simulink model "Scenario_MinimumExample_TwithTrafficLights_tol"  (R2021a)
settings: Solver=VariableStepAuto  StartTime=0.0  StopTime=50  RelTol=1e-3
model workspace (MAT data in the model file):
  Kz_dif : Simulink.Parameter (value not decoded)
  Kz_il : Simulink.Parameter (value not decoded)
  Kz_ir : Simulink.Parameter (value not decoded)
  Kz_is : Simulink.Parameter (value not decoded)
  Kz_long : Simulink.Parameter (value not decoded)
  Kz_pre : Simulink.Parameter (value not decoded)
  L_dif : Simulink.Parameter (value not decoded)
  L_il : Simulink.Parameter (value not decoded)
  L_ir : Simulink.Parameter (value not decoded)
  L_is : Simulink.Parameter (value not decoded)
  L_long : Simulink.Parameter (value not decoded)
  L_pre : Simulink.Parameter (value not decoded)
  Lc : Simulink.Parameter (value not decoded)
  Rk : Simulink.Parameter (value not decoded)
  Tz_dif : Simulink.Parameter (value not decoded)
  Tz_il : Simulink.Parameter (value not decoded)
  Tz_ir : Simulink.Parameter (value not decoded)
  Tz_is : Simulink.Parameter (value not decoded)
  Tz_long : Simulink.Parameter (value not decoded)
  Tz_pre : Simulink.Parameter (value not decoded)
  ds : Simulink.Parameter (value not decoded)
  dt : Simulink.Parameter (value not decoded)
  v : Simulink.Parameter (value not decoded)
symbols that are objects in the model workspace (value not decoded): Kz_dif, Kz_il, Kz_ir, Kz_is, Kz_long, Kz_pre, Rk, Tz_dif, Tz_il, Tz_ir, Tz_is, Tz_long, Tz_pre
libraries: StreetLanesLibrary x72, EdgesLibrary x64, MeasuringLibrary x33, SourcesAndSinksLibrary x12, LightsLibrary x2
(part 2 of 2)

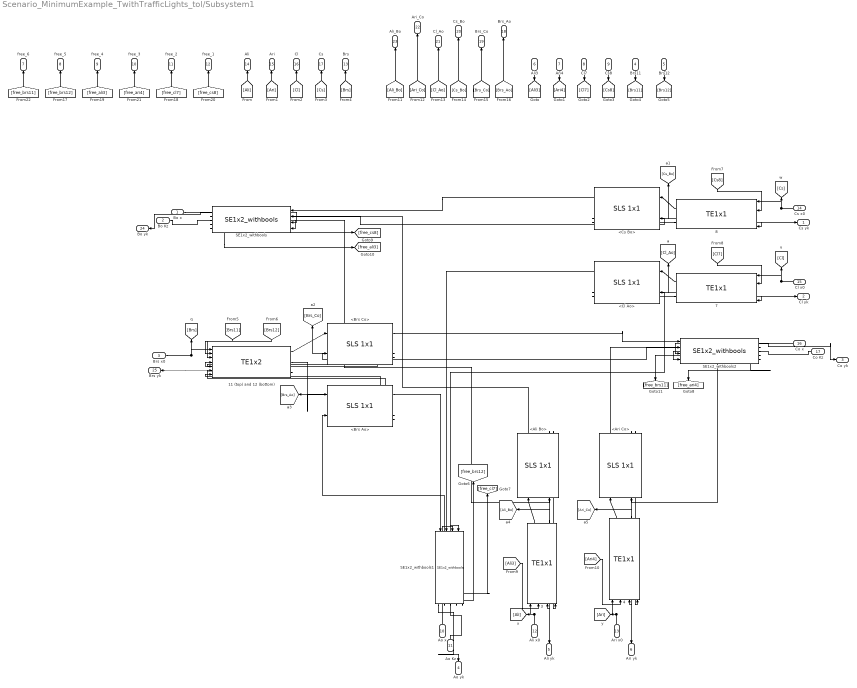
== system Scenario_MinimumExample_TwithTrafficLights_tol/Subsystem1 ==
  Bo x : Inport
  Bo Kz : Inport  Port=2
  Brs x0 : Inport  Port=3
  Brs11 : Inport  Port=4
  Brs12 : Inport  Port=5
  Ali3 : Inport  Port=6
  Ari4 : Inport  Port=7
  Cl7 : Inport  Port=8
  Cs8 : Inport  Port=9
  Ao x : Inport  Port=10
  Ao Kz : Inport  Port=11
  Ali x0 : Inport  Port=12
  Ari x0 : Inport  Port=13
  Cs x0 : Inport  Port=14
  Cl x0 : Inport  Port=15
  Co x : Inport  Port=16
  Co Kz : Inport  Port=17
  11 (top) and 12 (bottom) : EdgesLibrary/TE1x2  Rk1=0.5*Rk  Rk2=0.5*Rk
  {3..4,7..8} (4 alike) : EdgesLibrary/TE1x1  Rk=Rk  slope=2000
  <Ali Bo> : StreetLanesLibrary/SLS 1x1  Kz=Kz_left  Tz=Tz_left
  <Ari Co> : StreetLanesLibrary/SLS 1x1  Kz=Kz_right  Tz=Tz_right
  <Brs Ao> : StreetLanesLibrary/SLS 1x1  Kz=Kz_right  Tz=Tz_right
  <Brs Co> : StreetLanesLibrary/SLS 1x1  Kz=Kz_straight  Tz=Tz_straight
  <Cl Ao> : StreetLanesLibrary/SLS 1x1  Kz=Kz_left  Tz=Tz_left
  <Cs Bo> : StreetLanesLibrary/SLS 1x1  Kz=Kz_straight  Tz=Tz_straight
  SE1x2_withbools : EdgesLibrary/SE1x2_withbools  Rk1=Rk  Rk2=Rk
  SE1x2_withbools1 : EdgesLibrary/SE1x2_withbools  Rk1=Rk  Rk2=Rk
  SE1x2_withbools2 : EdgesLibrary/SE1x2_withbools  Rk1=Rk  Rk2=Rk
  Cs yk : Outport
  Cl yk : Outport  Port=2
  Co yk : Outport  Port=3
  Ao yk : Outport  Port=4
  Ali yk : Outport  Port=5
  Ari yk : Outport  Port=6
  free_6 : Outport  Port=7
  free_5 : Outport  Port=8
  free_4 : Outport  Port=9
  free_3 : Outport  Port=10
  free_2 : Outport  Port=11
  free_1 : Outport  Port=12
  Brs : Outport  Port=13
  Ali : Outport  Port=14
  Ari : Outport  Port=15
  Cl : Outport  Port=16
  Cs : Outport  Port=17
  Brs_Ao : Outport  Port=18
  Brs_Co : Outport  Port=19
  Cs_Bo : Outport  Port=20
  Cl_Ao : Outport  Port=21
  Ari_Co : Outport  Port=22
  Ali_Bo : Outport  Port=23
  Bo yk : Outport  Port=24
  Brs yk : Outport  Port=25
  wires:
  11 (top) and 12 (bottom)/2 -> <Brs Ao>/1
  11 (top) and 12 (bottom)/3 -> Brs yk/1
  3/2 -> Ali yk/1
  3/1 -> <Ali Bo>/1
  Ari x0/1 -> [Ari], 4/1
  <Cs Bo>/2 -> SE1x2_withbools/1
  <Cs Bo>/8 -> 8/4
  <Cl Ao>/8 -> 7/4
  Co x/1 -> SE1x2_withbools2/3
  SE1x2_withbools2/1 -> Co yk/1
  SE1x2_withbools2/3 -> <Ari Co>/2
  <Ari Co>/8 -> 4/4
  <Ali Bo>/8 -> 3/4
  Ao x/1 -> SE1x2_withbools1/3
  Brs x0/1 -> 11 (top) and 12 (bottom)/1, [Brs]
  <Brs Co>/2 -> SE1x2_withbools2/1
  <Cl Ao>/7 -> [Cl_Ao], 7/3
  <Cl Ao>/2 -> SE1x2_withbools1/2
  SE1x2_withbools/2 -> <Cs Bo>/2
  <Ari Co>/2 -> SE1x2_withbools2/2
  7/1 -> <Cl Ao>/1
  Cl x0/1 -> [Cl], 7/1
  4/1 -> <Ari Co>/1
  <Ari Co>/7 -> 4/3, [Ari_Co]
  <Brs Ao>/2 -> SE1x2_withbools1/1
  Ao Kz/1 -> SE1x2_withbools1/4
  <Brs Ao>/7 -> [Brs_Ao], 11 (top) and 12 (bottom)/6
  <Brs Ao>/8 -> 11 (top) and 12 (bottom)/7
  Co Kz/1 -> SE1x2_withbools2/4
  8/2 -> Cs yk/1
  Bo Kz/1 -> SE1x2_withbools/4
  SE1x2_withbools1/3 -> <Cl Ao>/2
  <Brs Co>/8 -> 11 (top) and 12 (bottom)/5
  [Brs12] -> 11 (top) and 12 (bottom)/3
  SE1x2_withbools/3 -> <Ali Bo>/2
  <Ali Bo>/7 -> 3/3, [Ali_Bo]
  SE1x2_withbools1/2 -> <Brs Ao>/2
  Ali x0/1 -> [Ali], 3/1
  <Brs Co>/7 -> 11 (top) and 12 (bottom)/4, [Brs_Co]
  SE1x2_withbools1/1 -> Ao yk/1
  <Ali Bo>/2 -> SE1x2_withbools/2
  [Ari4] -> 4/2
  SE1x2_withbools2/2 -> <Brs Co>/2
  8/1 -> <Cs Bo>/1
  4/2 -> Ari yk/1
  <Cs Bo>/7 -> 8/3, [Cs_Bo]
  Cs x0/1 -> [Cs], 8/1
  [Ali3] -> 3/2
  [Brs11] -> 11 (top) and 12 (bottom)/2
  11 (top) and 12 (bottom)/1 -> <Brs Co>/1
  Bo x/1 -> SE1x2_withbools/3
  [Cl7] -> 7/2
  SE1x2_withbools/1 -> Bo yk/1
  7/2 -> Cl yk/1
  [Cs8] -> 8/2
  [Ali_Bo] -> Ali_Bo/1
  [Ari_Co] -> Ari_Co/1
  [Cl_Ao] -> Cl_Ao/1
  [Cs_Bo] -> Cs_Bo/1
  [Brs_Co] -> Brs_Co/1
  [Brs_Ao] -> Brs_Ao/1
  [Ali] -> Ali/1
  [Ari] -> Ari/1
  [Cl] -> Cl/1
  [Cs] -> Cs/1
  [Brs] -> Brs/1
  Ali3/1 -> [Ali3]
  Ari4/1 -> [Ari4]
  Cl7/1 -> [Cl7]
  Cs8/1 -> [Cs8]
  Brs11/1 -> [Brs11]
  Brs12/1 -> [Brs12]
  SE1x2_withbools1/4 -> [free_brs12]
  SE1x2_withbools1/5 -> [free_cl7]
  SE1x2_withbools/4 -> [free_cs8]
  SE1x2_withbools/5 -> [free_ali3]
  SE1x2_withbools2/5 -> [free_ari4]
  SE1x2_withbools2/4 -> [free_brs11]
  [free_cs8] -> free_1/1
  [free_cl7] -> free_2/1
  [free_ari4] -> free_3/1
  [free_ali3] -> free_4/1
  [free_brs12] -> free_5/1
  [free_brs11] -> free_6/1

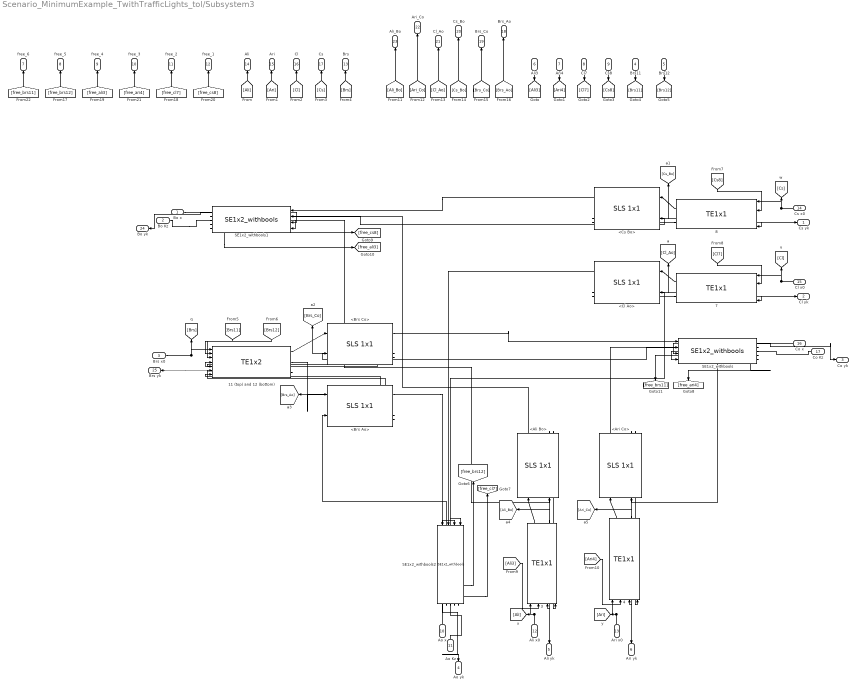
== system Scenario_MinimumExample_TwithTrafficLights_tol/Subsystem3 ==
  Bo x : Inport
  Bo Kz : Inport  Port=2
  Brs x0 : Inport  Port=3
  Brs11 : Inport  Port=4
  Brs12 : Inport  Port=5
  Ali3 : Inport  Port=6
  Ari4 : Inport  Port=7
  Cl7 : Inport  Port=8
  Cs8 : Inport  Port=9
  Ao x : Inport  Port=10
  Ao Kz : Inport  Port=11
  Ali x0 : Inport  Port=12
  Ari x0 : Inport  Port=13
  Cs x0 : Inport  Port=14
  Cl x0 : Inport  Port=15
  Co x : Inport  Port=16
  Co Kz : Inport  Port=17
  11 (top) and 12 (bottom) : EdgesLibrary/TE1x2  Rk1=0.5*Rk  Rk2=0.5*Rk
  {3..4,7..8} (4 alike) : EdgesLibrary/TE1x1  Rk=Rk  slope=2000
  <Ali Bo> : StreetLanesLibrary/SLS 1x1  Kz=Kz_left  Tz=Tz_left
  <Ari Co> : StreetLanesLibrary/SLS 1x1  Kz=Kz_right  Tz=Tz_right
  <Brs Ao> : StreetLanesLibrary/SLS 1x1  Kz=Kz_right  Tz=Tz_right
  <Brs Co> : StreetLanesLibrary/SLS 1x1  Kz=Kz_straight  Tz=Tz_straight
  <Cl Ao> : StreetLanesLibrary/SLS 1x1  Kz=Kz_left  Tz=Tz_left
  <Cs Bo> : StreetLanesLibrary/SLS 1x1  Kz=Kz_straight  Tz=Tz_straight
  SE1x2_withbools : EdgesLibrary/SE1x2_withbools  Rk1=Rk  Rk2=Rk
  SE1x2_withbools1 : EdgesLibrary/SE1x2_withbools  Rk1=Rk  Rk2=Rk
  SE1x2_withbools2 : EdgesLibrary/SE1x2_withbools  Rk1=Rk  Rk2=Rk
  Cs yk : Outport
  Cl yk : Outport  Port=2
  Co yk : Outport  Port=3
  Ao yk : Outport  Port=4
  Ali yk : Outport  Port=5
  Ari yk : Outport  Port=6
  free_6 : Outport  Port=7
  free_5 : Outport  Port=8
  free_4 : Outport  Port=9
  free_3 : Outport  Port=10
  free_2 : Outport  Port=11
  free_1 : Outport  Port=12
  Brs : Outport  Port=13
  Ali : Outport  Port=14
  Ari : Outport  Port=15
  Cl : Outport  Port=16
  Cs : Outport  Port=17
  Brs_Ao : Outport  Port=18
  Brs_Co : Outport  Port=19
  Cs_Bo : Outport  Port=20
  Cl_Ao : Outport  Port=21
  Ari_Co : Outport  Port=22
  Ali_Bo : Outport  Port=23
  Bo yk : Outport  Port=24
  Brs yk : Outport  Port=25
  wires:
  11 (top) and 12 (bottom)/2 -> <Brs Ao>/1
  11 (top) and 12 (bottom)/3 -> Brs yk/1
  3/2 -> Ali yk/1
  3/1 -> <Ali Bo>/1
  Ari x0/1 -> [Ari], 4/1
  <Cs Bo>/2 -> SE1x2_withbools1/1
  <Cs Bo>/8 -> 8/4
  <Cl Ao>/8 -> 7/4
  Co x/1 -> SE1x2_withbools/3
  SE1x2_withbools/1 -> Co yk/1
  SE1x2_withbools/3 -> <Ari Co>/2
  <Ari Co>/8 -> 4/4
  <Ali Bo>/8 -> 3/4
  Ao x/1 -> SE1x2_withbools2/3
  Brs x0/1 -> 11 (top) and 12 (bottom)/1, [Brs]
  <Brs Co>/2 -> SE1x2_withbools/1
  <Cl Ao>/7 -> [Cl_Ao], 7/3
  <Cl Ao>/2 -> SE1x2_withbools2/2
  SE1x2_withbools1/2 -> <Cs Bo>/2
  <Ari Co>/2 -> SE1x2_withbools/2
  7/1 -> <Cl Ao>/1
  Cl x0/1 -> [Cl], 7/1
  4/1 -> <Ari Co>/1
  <Ari Co>/7 -> 4/3, [Ari_Co]
  <Brs Ao>/2 -> SE1x2_withbools2/1
  Ao Kz/1 -> SE1x2_withbools2/4
  <Brs Ao>/7 -> [Brs_Ao], 11 (top) and 12 (bottom)/6
  <Brs Ao>/8 -> 11 (top) and 12 (bottom)/7
  Co Kz/1 -> SE1x2_withbools/4
  8/2 -> Cs yk/1
  Bo Kz/1 -> SE1x2_withbools1/4
  SE1x2_withbools2/3 -> <Cl Ao>/2
  <Brs Co>/8 -> 11 (top) and 12 (bottom)/5
  [Brs12] -> 11 (top) and 12 (bottom)/3
  SE1x2_withbools1/3 -> <Ali Bo>/2
  <Ali Bo>/7 -> 3/3, [Ali_Bo]
  SE1x2_withbools2/2 -> <Brs Ao>/2
  Ali x0/1 -> [Ali], 3/1
  <Brs Co>/7 -> 11 (top) and 12 (bottom)/4, [Brs_Co]
  SE1x2_withbools2/1 -> Ao yk/1
  <Ali Bo>/2 -> SE1x2_withbools1/2
  [Ari4] -> 4/2
  SE1x2_withbools/2 -> <Brs Co>/2
  8/1 -> <Cs Bo>/1
  4/2 -> Ari yk/1
  <Cs Bo>/7 -> 8/3, [Cs_Bo]
  Cs x0/1 -> [Cs], 8/1
  [Ali3] -> 3/2
  [Brs11] -> 11 (top) and 12 (bottom)/2
  11 (top) and 12 (bottom)/1 -> <Brs Co>/1
  Bo x/1 -> SE1x2_withbools1/3
  [Cl7] -> 7/2
  SE1x2_withbools1/1 -> Bo yk/1
  7/2 -> Cl yk/1
  [Cs8] -> 8/2
  [Ali_Bo] -> Ali_Bo/1
  [Ari_Co] -> Ari_Co/1
  [Cl_Ao] -> Cl_Ao/1
  [Cs_Bo] -> Cs_Bo/1
  [Brs_Co] -> Brs_Co/1
  [Brs_Ao] -> Brs_Ao/1
  [Ali] -> Ali/1
  [Ari] -> Ari/1
  [Cl] -> Cl/1
  [Cs] -> Cs/1
  [Brs] -> Brs/1
  Ali3/1 -> [Ali3]
  Ari4/1 -> [Ari4]
  Cl7/1 -> [Cl7]
  Cs8/1 -> [Cs8]
  Brs11/1 -> [Brs11]
  Brs12/1 -> [Brs12]
  SE1x2_withbools2/4 -> [free_brs12]
  SE1x2_withbools2/5 -> [free_cl7]
  SE1x2_withbools1/4 -> [free_cs8]
  SE1x2_withbools1/5 -> [free_ali3]
  SE1x2_withbools/5 -> [free_ari4]
  SE1x2_withbools/4 -> [free_brs11]
  [free_cs8] -> free_1/1
  [free_cl7] -> free_2/1
  [free_ari4] -> free_3/1
  [free_ali3] -> free_4/1
  [free_brs12] -> free_5/1
  [free_brs11] -> free_6/1

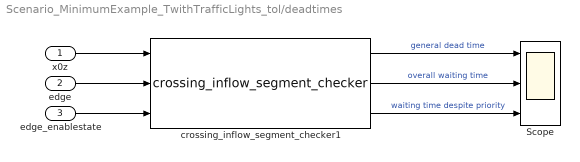
== system Scenario_MinimumExample_TwithTrafficLights_tol/deadtimes ==
  x0z : Inport
  edge : Inport  Port=2
  edge_enablestate : Inport  Port=3
  Scope : Scope  NumInputPorts=3
  crossing_inflow_segment_checker1 : MeasuringLibrary/crossing_inflow_segment_checker  SystemSampleTime=-1  VariantActivationTime=update diagram  Latency=0  AutoFrameSizeCalculation=off
  wires:
  crossing_inflow_segment_checker1/3 -> Scope/3  "waiting time despite priority"
  x0z/1 -> crossing_inflow_segment_checker1/1
  edge/1 -> crossing_inflow_segment_checker1/2
  crossing_inflow_segment_checker1/2 -> Scope/2  "overall waiting time"
  edge_enablestate/1 -> crossing_inflow_segment_checker1/3
  crossing_inflow_segment_checker1/1 -> Scope/1  "general dead time"

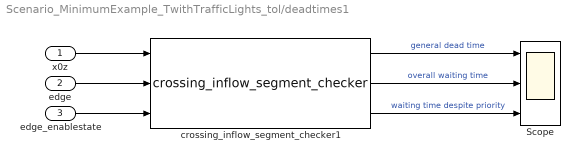
== system Scenario_MinimumExample_TwithTrafficLights_tol/deadtimes1 ==
  x0z : Inport
  edge : Inport  Port=2
  edge_enablestate : Inport  Port=3
  Scope : Scope  NumInputPorts=3
  crossing_inflow_segment_checker1 : MeasuringLibrary/crossing_inflow_segment_checker  SystemSampleTime=-1  VariantActivationTime=update diagram  Latency=0  AutoFrameSizeCalculation=off
  wires:
  crossing_inflow_segment_checker1/3 -> Scope/3  "waiting time despite priority"
  x0z/1 -> crossing_inflow_segment_checker1/1
  edge/1 -> crossing_inflow_segment_checker1/2
  crossing_inflow_segment_checker1/2 -> Scope/2  "overall waiting time"
  edge_enablestate/1 -> crossing_inflow_segment_checker1/3
  crossing_inflow_segment_checker1/1 -> Scope/1  "general dead time"

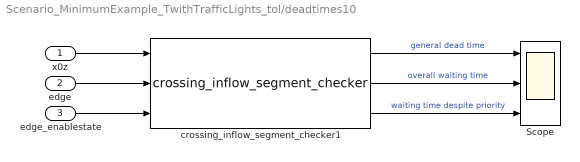
== system Scenario_MinimumExample_TwithTrafficLights_tol/deadtimes10 ==
  x0z : Inport
  edge : Inport  Port=2
  edge_enablestate : Inport  Port=3
  Scope : Scope  NumInputPorts=3
  crossing_inflow_segment_checker1 : MeasuringLibrary/crossing_inflow_segment_checker  SystemSampleTime=-1  VariantActivationTime=update diagram  Latency=0  AutoFrameSizeCalculation=off
  wires:
  crossing_inflow_segment_checker1/3 -> Scope/3  "waiting time despite priority"
  x0z/1 -> crossing_inflow_segment_checker1/1
  edge/1 -> crossing_inflow_segment_checker1/2
  crossing_inflow_segment_checker1/2 -> Scope/2  "overall waiting time"
  edge_enablestate/1 -> crossing_inflow_segment_checker1/3
  crossing_inflow_segment_checker1/1 -> Scope/1  "general dead time"

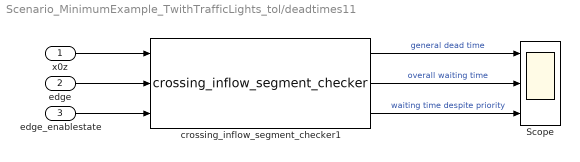
== system Scenario_MinimumExample_TwithTrafficLights_tol/deadtimes11 ==
  x0z : Inport
  edge : Inport  Port=2
  edge_enablestate : Inport  Port=3
  Scope : Scope  NumInputPorts=3
  crossing_inflow_segment_checker1 : MeasuringLibrary/crossing_inflow_segment_checker  SystemSampleTime=-1  VariantActivationTime=update diagram  Latency=0  AutoFrameSizeCalculation=off
  wires:
  crossing_inflow_segment_checker1/3 -> Scope/3  "waiting time despite priority"
  x0z/1 -> crossing_inflow_segment_checker1/1
  edge/1 -> crossing_inflow_segment_checker1/2
  crossing_inflow_segment_checker1/2 -> Scope/2  "overall waiting time"
  edge_enablestate/1 -> crossing_inflow_segment_checker1/3
  crossing_inflow_segment_checker1/1 -> Scope/1  "general dead time"

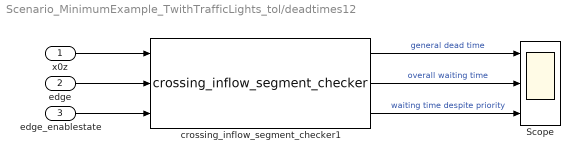
== system Scenario_MinimumExample_TwithTrafficLights_tol/deadtimes12 ==
  x0z : Inport
  edge : Inport  Port=2
  edge_enablestate : Inport  Port=3
  Scope : Scope  NumInputPorts=3
  crossing_inflow_segment_checker1 : MeasuringLibrary/crossing_inflow_segment_checker  SystemSampleTime=-1  VariantActivationTime=update diagram  Latency=0  AutoFrameSizeCalculation=off
  wires:
  crossing_inflow_segment_checker1/3 -> Scope/3  "waiting time despite priority"
  x0z/1 -> crossing_inflow_segment_checker1/1
  edge/1 -> crossing_inflow_segment_checker1/2
  crossing_inflow_segment_checker1/2 -> Scope/2  "overall waiting time"
  edge_enablestate/1 -> crossing_inflow_segment_checker1/3
  crossing_inflow_segment_checker1/1 -> Scope/1  "general dead time"

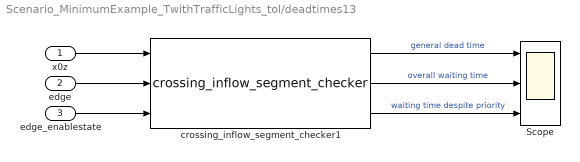
== system Scenario_MinimumExample_TwithTrafficLights_tol/deadtimes13 ==
  x0z : Inport
  edge : Inport  Port=2
  edge_enablestate : Inport  Port=3
  Scope : Scope  NumInputPorts=3
  crossing_inflow_segment_checker1 : MeasuringLibrary/crossing_inflow_segment_checker  SystemSampleTime=-1  VariantActivationTime=update diagram  Latency=0  AutoFrameSizeCalculation=off
  wires:
  crossing_inflow_segment_checker1/3 -> Scope/3  "waiting time despite priority"
  x0z/1 -> crossing_inflow_segment_checker1/1
  edge/1 -> crossing_inflow_segment_checker1/2
  crossing_inflow_segment_checker1/2 -> Scope/2  "overall waiting time"
  edge_enablestate/1 -> crossing_inflow_segment_checker1/3
  crossing_inflow_segment_checker1/1 -> Scope/1  "general dead time"

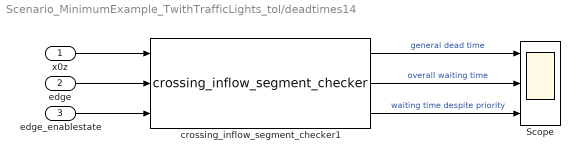
== system Scenario_MinimumExample_TwithTrafficLights_tol/deadtimes14 ==
  x0z : Inport
  edge : Inport  Port=2
  edge_enablestate : Inport  Port=3
  Scope : Scope  NumInputPorts=3
  crossing_inflow_segment_checker1 : MeasuringLibrary/crossing_inflow_segment_checker  SystemSampleTime=-1  VariantActivationTime=update diagram  Latency=0  AutoFrameSizeCalculation=off
  wires:
  crossing_inflow_segment_checker1/3 -> Scope/3  "waiting time despite priority"
  x0z/1 -> crossing_inflow_segment_checker1/1
  edge/1 -> crossing_inflow_segment_checker1/2
  crossing_inflow_segment_checker1/2 -> Scope/2  "overall waiting time"
  edge_enablestate/1 -> crossing_inflow_segment_checker1/3
  crossing_inflow_segment_checker1/1 -> Scope/1  "general dead time"

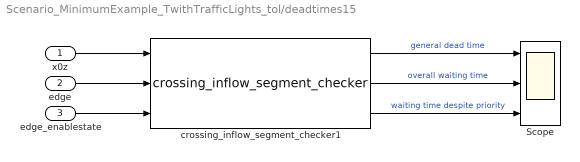
== system Scenario_MinimumExample_TwithTrafficLights_tol/deadtimes15 ==
  x0z : Inport
  edge : Inport  Port=2
  edge_enablestate : Inport  Port=3
  Scope : Scope  NumInputPorts=3
  crossing_inflow_segment_checker1 : MeasuringLibrary/crossing_inflow_segment_checker  SystemSampleTime=-1  VariantActivationTime=update diagram  Latency=0  AutoFrameSizeCalculation=off
  wires:
  crossing_inflow_segment_checker1/3 -> Scope/3  "waiting time despite priority"
  x0z/1 -> crossing_inflow_segment_checker1/1
  edge/1 -> crossing_inflow_segment_checker1/2
  crossing_inflow_segment_checker1/2 -> Scope/2  "overall waiting time"
  edge_enablestate/1 -> crossing_inflow_segment_checker1/3
  crossing_inflow_segment_checker1/1 -> Scope/1  "general dead time"

== system Scenario_MinimumExample_TwithTrafficLights_tol/deadtimes16 ==
  x0z : Inport
  edge : Inport  Port=2
  edge_enablestate : Inport  Port=3
  Scope : Scope  NumInputPorts=3
  crossing_inflow_segment_checker1 : MeasuringLibrary/crossing_inflow_segment_checker  SystemSampleTime=-1  VariantActivationTime=update diagram  Latency=0  AutoFrameSizeCalculation=off
  wires:
  crossing_inflow_segment_checker1/3 -> Scope/3  "waiting time despite priority"
  x0z/1 -> crossing_inflow_segment_checker1/1
  edge/1 -> crossing_inflow_segment_checker1/2
  crossing_inflow_segment_checker1/2 -> Scope/2  "overall waiting time"
  edge_enablestate/1 -> crossing_inflow_segment_checker1/3
  crossing_inflow_segment_checker1/1 -> Scope/1  "general dead time"

== system Scenario_MinimumExample_TwithTrafficLights_tol/deadtimes17 ==
  x0z : Inport
  edge : Inport  Port=2
  edge_enablestate : Inport  Port=3
  Scope : Scope  NumInputPorts=3
  crossing_inflow_segment_checker1 : MeasuringLibrary/crossing_inflow_segment_checker  SystemSampleTime=-1  VariantActivationTime=update diagram  Latency=0  AutoFrameSizeCalculation=off
  wires:
  crossing_inflow_segment_checker1/3 -> Scope/3  "waiting time despite priority"
  x0z/1 -> crossing_inflow_segment_checker1/1
  edge/1 -> crossing_inflow_segment_checker1/2
  crossing_inflow_segment_checker1/2 -> Scope/2  "overall waiting time"
  edge_enablestate/1 -> crossing_inflow_segment_checker1/3
  crossing_inflow_segment_checker1/1 -> Scope/1  "general dead time"

== system Scenario_MinimumExample_TwithTrafficLights_tol/deadtimes2 ==
  x0z : Inport
  edge : Inport  Port=2
  edge_enablestate : Inport  Port=3
  Scope : Scope  NumInputPorts=3
  crossing_inflow_segment_checker1 : MeasuringLibrary/crossing_inflow_segment_checker  SystemSampleTime=-1  VariantActivationTime=update diagram  Latency=0  AutoFrameSizeCalculation=off
  wires:
  crossing_inflow_segment_checker1/3 -> Scope/3  "waiting time despite priority"
  x0z/1 -> crossing_inflow_segment_checker1/1
  edge/1 -> crossing_inflow_segment_checker1/2
  crossing_inflow_segment_checker1/2 -> Scope/2  "overall waiting time"
  edge_enablestate/1 -> crossing_inflow_segment_checker1/3
  crossing_inflow_segment_checker1/1 -> Scope/1  "general dead time"

== system Scenario_MinimumExample_TwithTrafficLights_tol/deadtimes3 ==
  x0z : Inport
  edge : Inport  Port=2
  edge_enablestate : Inport  Port=3
  Scope : Scope  NumInputPorts=3
  crossing_inflow_segment_checker1 : MeasuringLibrary/crossing_inflow_segment_checker  SystemSampleTime=-1  VariantActivationTime=update diagram  Latency=0  AutoFrameSizeCalculation=off
  wires:
  crossing_inflow_segment_checker1/3 -> Scope/3  "waiting time despite priority"
  x0z/1 -> crossing_inflow_segment_checker1/1
  edge/1 -> crossing_inflow_segment_checker1/2
  crossing_inflow_segment_checker1/2 -> Scope/2  "overall waiting time"
  edge_enablestate/1 -> crossing_inflow_segment_checker1/3
  crossing_inflow_segment_checker1/1 -> Scope/1  "general dead time"

== system Scenario_MinimumExample_TwithTrafficLights_tol/deadtimes4 ==
  x0z : Inport
  edge : Inport  Port=2
  edge_enablestate : Inport  Port=3
  Scope : Scope  NumInputPorts=3
  crossing_inflow_segment_checker1 : MeasuringLibrary/crossing_inflow_segment_checker  SystemSampleTime=-1  VariantActivationTime=update diagram  Latency=0  AutoFrameSizeCalculation=off
  wires:
  crossing_inflow_segment_checker1/3 -> Scope/3  "waiting time despite priority"
  x0z/1 -> crossing_inflow_segment_checker1/1
  edge/1 -> crossing_inflow_segment_checker1/2
  crossing_inflow_segment_checker1/2 -> Scope/2  "overall waiting time"
  edge_enablestate/1 -> crossing_inflow_segment_checker1/3
  crossing_inflow_segment_checker1/1 -> Scope/1  "general dead time"

== system Scenario_MinimumExample_TwithTrafficLights_tol/deadtimes5 ==
  x0z : Inport
  edge : Inport  Port=2
  edge_enablestate : Inport  Port=3
  Scope : Scope  NumInputPorts=3
  crossing_inflow_segment_checker1 : MeasuringLibrary/crossing_inflow_segment_checker  SystemSampleTime=-1  VariantActivationTime=update diagram  Latency=0  AutoFrameSizeCalculation=off
  wires:
  crossing_inflow_segment_checker1/3 -> Scope/3  "waiting time despite priority"
  x0z/1 -> crossing_inflow_segment_checker1/1
  edge/1 -> crossing_inflow_segment_checker1/2
  crossing_inflow_segment_checker1/2 -> Scope/2  "overall waiting time"
  edge_enablestate/1 -> crossing_inflow_segment_checker1/3
  crossing_inflow_segment_checker1/1 -> Scope/1  "general dead time"

== system Scenario_MinimumExample_TwithTrafficLights_tol/deadtimes6 ==
  x0z : Inport
  edge : Inport  Port=2
  edge_enablestate : Inport  Port=3
  Scope : Scope  NumInputPorts=3
  crossing_inflow_segment_checker1 : MeasuringLibrary/crossing_inflow_segment_checker  SystemSampleTime=-1  VariantActivationTime=update diagram  Latency=0  AutoFrameSizeCalculation=off
  wires:
  crossing_inflow_segment_checker1/3 -> Scope/3  "waiting time despite priority"
  x0z/1 -> crossing_inflow_segment_checker1/1
  edge/1 -> crossing_inflow_segment_checker1/2
  crossing_inflow_segment_checker1/2 -> Scope/2  "overall waiting time"
  edge_enablestate/1 -> crossing_inflow_segment_checker1/3
  crossing_inflow_segment_checker1/1 -> Scope/1  "general dead time"

== system Scenario_MinimumExample_TwithTrafficLights_tol/deadtimes7 ==
  x0z : Inport
  edge : Inport  Port=2
  edge_enablestate : Inport  Port=3
  Scope : Scope  NumInputPorts=3
  crossing_inflow_segment_checker1 : MeasuringLibrary/crossing_inflow_segment_checker  SystemSampleTime=-1  VariantActivationTime=update diagram  Latency=0  AutoFrameSizeCalculation=off
  wires:
  crossing_inflow_segment_checker1/3 -> Scope/3  "waiting time despite priority"
  x0z/1 -> crossing_inflow_segment_checker1/1
  edge/1 -> crossing_inflow_segment_checker1/2
  crossing_inflow_segment_checker1/2 -> Scope/2  "overall waiting time"
  edge_enablestate/1 -> crossing_inflow_segment_checker1/3
  crossing_inflow_segment_checker1/1 -> Scope/1  "general dead time"

== system Scenario_MinimumExample_TwithTrafficLights_tol/deadtimes8 ==
  x0z : Inport
  edge : Inport  Port=2
  edge_enablestate : Inport  Port=3
  Scope : Scope  NumInputPorts=3
  crossing_inflow_segment_checker1 : MeasuringLibrary/crossing_inflow_segment_checker  SystemSampleTime=-1  VariantActivationTime=update diagram  Latency=0  AutoFrameSizeCalculation=off
  wires:
  crossing_inflow_segment_checker1/3 -> Scope/3  "waiting time despite priority"
  x0z/1 -> crossing_inflow_segment_checker1/1
  edge/1 -> crossing_inflow_segment_checker1/2
  crossing_inflow_segment_checker1/2 -> Scope/2  "overall waiting time"
  edge_enablestate/1 -> crossing_inflow_segment_checker1/3
  crossing_inflow_segment_checker1/1 -> Scope/1  "general dead time"

== system Scenario_MinimumExample_TwithTrafficLights_tol/deadtimes9 ==
  x0z : Inport
  edge : Inport  Port=2
  edge_enablestate : Inport  Port=3
  Scope : Scope  NumInputPorts=3
  crossing_inflow_segment_checker1 : MeasuringLibrary/crossing_inflow_segment_checker  SystemSampleTime=-1  VariantActivationTime=update diagram  Latency=0  AutoFrameSizeCalculation=off
  wires:
  crossing_inflow_segment_checker1/3 -> Scope/3  "waiting time despite priority"
  x0z/1 -> crossing_inflow_segment_checker1/1
  edge/1 -> crossing_inflow_segment_checker1/2
  crossing_inflow_segment_checker1/2 -> Scope/2  "overall waiting time"
  edge_enablestate/1 -> crossing_inflow_segment_checker1/3
  crossing_inflow_segment_checker1/1 -> Scope/1  "general dead time"

== system Scenario_MinimumExample_TwithTrafficLights_tol/rel xz ==
  xz : Inport
  kz : Inport  Port=2
  Scope : Scope
  rel xz1 : MeasuringLibrary/rel xz  SystemSampleTime=-1  VariantActivationTime=update diagram  Latency=0  AutoFrameSizeCalculation=off
  wires:
  xz/1 -> rel xz1/1
  rel xz1/1 -> Scope/1  "relative xz"
  kz/1 -> rel xz1/2

== system Scenario_MinimumExample_TwithTrafficLights_tol/sinks ==
  edge : Inport
  Scope : Scope  NumInputPorts=2
  sink_edge_checker1 : MeasuringLibrary/sink_edge_checker  shortestPathTz=0
  wires:
  sink_edge_checker1/1 -> Scope/1  "maximum outflow time"
  edge/1 -> sink_edge_checker1/1
  sink_edge_checker1/2 -> Scope/2  "actual outflow time"

== system Scenario_MinimumExample_TwithTrafficLights_tol/sinks1 ==
  edge : Inport
  Scope : Scope  NumInputPorts=2
  sink_edge_checker1 : MeasuringLibrary/sink_edge_checker  shortestPathTz=shortestPathTz
  wires:
  sink_edge_checker1/1 -> Scope/1  "maximum outflow time"
  edge/1 -> sink_edge_checker1/1
  sink_edge_checker1/2 -> Scope/2  "actual outflow time"

== system Scenario_MinimumExample_TwithTrafficLights_tol/sinks2 ==
  edge : Inport
  Scope : Scope  NumInputPorts=2
  sink_edge_checker1 : MeasuringLibrary/sink_edge_checker  shortestPathTz=shortestPathTz
  wires:
  sink_edge_checker1/1 -> Scope/1  "maximum outflow time"
  edge/1 -> sink_edge_checker1/1
  sink_edge_checker1/2 -> Scope/2  "actual outflow time"

== system Scenario_MinimumExample_TwithTrafficLights_tol/sinks3 ==
  edge : Inport
  Scope : Scope  NumInputPorts=2
  sink_edge_checker1 : MeasuringLibrary/sink_edge_checker  shortestPathTz=shortestPathTz
  wires:
  sink_edge_checker1/1 -> Scope/1  "maximum outflow time"
  edge/1 -> sink_edge_checker1/1
  sink_edge_checker1/2 -> Scope/2  "actual outflow time"

== system Scenario_MinimumExample_TwithTrafficLights_tol/sinks4 ==
  edge : Inport
  Scope : Scope  NumInputPorts=2
  sink_edge_checker1 : MeasuringLibrary/sink_edge_checker  shortestPathTz=shortestPathTz
  wires:
  sink_edge_checker1/1 -> Scope/1  "maximum outflow time"
  edge/1 -> sink_edge_checker1/1
  sink_edge_checker1/2 -> Scope/2  "actual outflow time"

== system Scenario_MinimumExample_TwithTrafficLights_tol/sinks5 ==
  edge : Inport
  Scope : Scope  NumInputPorts=2
  sink_edge_checker1 : MeasuringLibrary/sink_edge_checker  shortestPathTz=shortestPathTz
  wires:
  sink_edge_checker1/1 -> Scope/1  "maximum outflow time"
  edge/1 -> sink_edge_checker1/1
  sink_edge_checker1/2 -> Scope/2  "actual outflow time"

== system Scenario_MinimumExample_TwithTrafficLights_tol/sinks6 ==
  edge : Inport
  Scope : Scope  NumInputPorts=2
  sink_edge_checker1 : MeasuringLibrary/sink_edge_checker  shortestPathTz=shortestPathTz
  wires:
  sink_edge_checker1/1 -> Scope/1  "maximum outflow time"
  edge/1 -> sink_edge_checker1/1
  sink_edge_checker1/2 -> Scope/2  "actual outflow time"

== system Scenario_MinimumExample_TwithTrafficLights_tol/sources ==
  edge : Inport
  Scope : Scope  NumInputPorts=2
  source_edge_checker1 : MeasuringLibrary/source_edge_checker  SystemSampleTime=-1  VariantActivationTime=update diagram  Latency=0  AutoFrameSizeCalculation=off
  wires:
  source_edge_checker1/1 -> Scope/1  "maximum inflow time"
  source_edge_checker1/2 -> Scope/2  "actual inflow time"
  edge/1 -> source_edge_checker1/1

== system Scenario_MinimumExample_TwithTrafficLights_tol/sources1 ==
  edge : Inport
  Scope : Scope  NumInputPorts=2
  source_edge_checker1 : MeasuringLibrary/source_edge_checker  SystemSampleTime=-1  VariantActivationTime=update diagram  Latency=0  AutoFrameSizeCalculation=off
  wires:
  source_edge_checker1/1 -> Scope/1  "maximum inflow time"
  source_edge_checker1/2 -> Scope/2  "actual inflow time"
  edge/1 -> source_edge_checker1/1

== system Scenario_MinimumExample_TwithTrafficLights_tol/sources2 ==
  edge : Inport
  Scope : Scope  NumInputPorts=2
  source_edge_checker1 : MeasuringLibrary/source_edge_checker  SystemSampleTime=-1  VariantActivationTime=update diagram  Latency=0  AutoFrameSizeCalculation=off
  wires:
  source_edge_checker1/1 -> Scope/1  "maximum inflow time"
  source_edge_checker1/2 -> Scope/2  "actual inflow time"
  edge/1 -> source_edge_checker1/1

== system Scenario_MinimumExample_TwithTrafficLights_tol/sources4 ==
  edge : Inport
  Scope : Scope  NumInputPorts=2
  source_edge_checker1 : MeasuringLibrary/source_edge_checker  SystemSampleTime=-1  VariantActivationTime=update diagram  Latency=0  AutoFrameSizeCalculation=off
  wires:
  source_edge_checker1/1 -> Scope/1  "maximum inflow time"
  source_edge_checker1/2 -> Scope/2  "actual inflow time"
  edge/1 -> source_edge_checker1/1

== system Scenario_MinimumExample_TwithTrafficLights_tol/sources5 ==
  edge : Inport
  Scope : Scope  NumInputPorts=2
  source_edge_checker1 : MeasuringLibrary/source_edge_checker  SystemSampleTime=-1  VariantActivationTime=update diagram  Latency=0  AutoFrameSizeCalculation=off
  wires:
  source_edge_checker1/1 -> Scope/1  "maximum inflow time"
  source_edge_checker1/2 -> Scope/2  "actual inflow time"
  edge/1 -> source_edge_checker1/1

== system Scenario_MinimumExample_TwithTrafficLights_tol/sources6 ==
  edge : Inport
  Scope : Scope  NumInputPorts=2
  source_edge_checker1 : MeasuringLibrary/source_edge_checker  SystemSampleTime=-1  VariantActivationTime=update diagram  Latency=0  AutoFrameSizeCalculation=off
  wires:
  source_edge_checker1/1 -> Scope/1  "maximum inflow time"
  source_edge_checker1/2 -> Scope/2  "actual inflow time"
  edge/1 -> source_edge_checker1/1

== stateflow chart Scenario_MinimumExample_TwithTrafficLights_tol/Plus-Controller ==
  note: ?
  state Group__Crs_Brs
  state Group__Cl_Bl
  state Group__Ars_Drs
  state Group__Al_Dl
  note: check
      | Crs straight
      | crossings
  note: check
      | Cl
      | crossings
  note: check
      | Ars straight
      | crossings
  note: check
      | Al
      | crossings
  note: check
      | Crs right
      | crossings
  note: check
      | Bl
      | crossings
  note: check
      | Ars right
      | crossings
  note: check
      | Dl
      | crossings
  note: check
      | Brs straight
      | crossings
  note: check
      | Drs straight
      | crossings
  note: check
      | Brs right
      | crossings
  note: check
      | Drs right
      | crossings
  Group__Al_Dl -> Group__Crs_Brs [order 2] : [[[after(green_duration_l, sec)]]]
      | {enAl = 0; enDl = 0;}
  Group__Ars_Drs -> Group__Al_Dl [order 1] : [[after(green_duration_sr, sec)]]
      | {enAs = 0; enAr = 0; enDs = 0; enDr = 0;}
  Group__Cl_Bl -> Group__Ars_Drs [order 1] : [after(green_duration_l, sec)]
      | {enCl = 0; enBl = 0;}
  Group__Crs_Brs -> Group__Cl_Bl [order 1] : [after(green_duration_sr, sec)]
      | {enCs = 0; enCr = 0; ...
      | enBs = 0; enBr = 0;}
  (default) -> Group__Crs_Brs : {enAl = 0; enAs = 0; enAr = 0;
      | enBl = 0; enBs = 0; enBr = 0;
      | enCl = 0; enCs = 0; enCr = 0;
      | enDl = 0; enDs = 0; enDr = 0;}
  Group__Crs_Brs -> (junction 51) [order 2]
  (junction 109) -> Group__Crs_Brs
  Group__Cl_Bl -> (junction 117) [order 2]
  (junction 126) -> Group__Cl_Bl
  Group__Ars_Drs -> (junction 134) [order 2]
  (junction 131) -> Group__Ars_Drs
  Group__Al_Dl -> (junction 151) [order 1]
  (junction 160) -> Group__Al_Dl
  (junction 117) -> (junction 116) [order 2] : {enCl = 0;}
  (junction 51) -> (junction 59) [order 1] : [(Dl_Co<=tol && Drs_Ao<=tol ...
      | && Drs_Bo<=tol && Bl_Do<=tol ...
      | && Al_Bo<=tol && Ars_Do<=tol)]
      | {enCs = 1;}
  (junction 117) -> (junction 116) [order 1] : [(Dl_Co<=tol && Drs_Ao<=tol && ....
      | Brs_Co<=tol && Al_Bo<=tol && ...
      | Ars_Do<=tol)]{enCl = 1;}
  (junction 51) -> (junction 59) [order 2] : {enCs = 0;}
  (junction 134) -> (junction 133) [order 1] : [((Cl_Ao<=tol && Crs_Bo<=tol && ...
      | Crs_Do<=tol && Dl_Co<=tol && ...
      | Bl_Do<=tol && Brs_Co<=tol))]
      | {enAs = 1;}
  (junction 151) -> (junction 150) [order 1] : [(Cl_Ao<=tol && Crs_Bo<=tol ...
      | && Drs_Ao<=tol && Bl_Do<=tol ...
      | && Brs_Co<=tol)]{enAl = 1;}
  (junction 134) -> (junction 133) [order 2] : {enAs = 0;}
  (junction 151) -> (junction 150) [order 2] : {enAl = 0;}
  (junction 59) -> (junction 104) [order 1] : [(Ars_Do<=tol && Bl_Do<=tol)]
      | {enCr = 1;}
  (junction 116) -> (junction 126) [order 1] : [(Al_Bo<=tol && Ars_Do<=tol && ...
      | Crs_Bo<=tol && Dl_Co<=tol && ...
      | Drs_Ao<=tol)]{enBl = 1;}
  (junction 59) -> (junction 104) [order 2] : {enCr = 0;}
  (junction 116) -> (junction 126) [order 2] : {enBl = 0;}
  (junction 133) -> (junction 143) [order 1] : [(Brs_Co<=tol && Dl_Co<=tol)]
      | {enAr = 1;}
  (junction 150) -> (junction 160) [order 1] : [(Bl_Do<=tol && Brs_Co<=tol ...
      | && Ars_Do<=tol && Cl_Ao<=tol ...
      | && Crs_Bo<=tol)]{enDl = 1;}
  (junction 133) -> (junction 143) [order 2] : {enAr = 0;}
  (junction 150) -> (junction 160) [order 2] : {enDl = 0;}
  (junction 104) -> (junction 105) [order 1] : [(Al_Bo<=tol && Ars_Do<=tol ...
      | && Ars_Co<=tol && Cl_Ao<=tol ...
      | && Dl_Co<=tol && Drs_Ao<=tol)]
      | {enBs = 1;}
  (junction 104) -> (junction 105) [order 2] : {enBs = 0;}
  (junction 143) -> (junction 141) [order 1] : [(Bl_Do<=tol && Brs_Co<=tol ...
      | && Brs_Ao<=tol && Al_Bo<=tol ...
      | && Cl_Ao<=tol && Crs_Bo<=tol)]
      | {enDs = 1;}
  (junction 143) -> (junction 141) [order 2] : {enDs=0;}
  (junction 105) -> (junction 109) [order 1] : [Drs_Ao<=tol && Cl_Ao<=tol]
      | {enBr = 1;}
  (junction 105) -> (junction 109) [order 2] : {enBr = 0;}
  (junction 141) -> (junction 131) [order 1] : [(Crs_Bo<=tol && Al_Bo<=tol)]
      | {enDr = 1;}
  (junction 141) -> (junction 131) [order 2] : {enDr = 0;}
  data: Bl input; Brs input; Al input; Ars input; Cl input; Crs input; Dl input; Drs input; Al_Bo input; Ars_Do input; Ars_Co input; Bl_Do input; Brs_Co input; Brs_Ao input; Cl_Ao input; Crs_Bo input; Crs_Do input; Dl_Co input; Drs_Ao input; Drs_Bo input; enAl output =0; enAs output =0; enAr output =0; enBl output =0; enBs output =0; enBr output =0; enCl output =0; enCs output =0; enCr output =0; enDl output =0; enDs output =0; enDr output =0; green_duration_sr parameter; green_duration_l parameter; tol parameter
